simulink model "pd_controller_j2n6s300"  (R2022a)
settings: Solver=ode4  StartTime=0.0  StopTime=0.2  FixedStep=0.01  RelTol=1e-3  EnableMultiTasking=on
undefined symbols (not defined in the file or in its folder): equation_of_motion
libraries: simulink x6
settings Model: Creator=user  LastModifiedBy=47116
settings SolverCC: AlgebraicLoopSolver=TrustRegion
settings DataIOCC: LimitDataPoints=on  SaveFormat=Array
settings OptimizationCC: LifeSpan=inf
settings DebuggingCC: UnconnectedInputMsg=warning  UnconnectedOutputMsg=warning  UnconnectedLineMsg=warning  SFUnexpectedBacktrackingDiag=warning  SFNoUnconditionalDefaultTransitionDiag=warning  SFExecutionAtInitializationDiag=none  SFMachineParentedDataDiag=warning  ArithmeticOperatorsInVariantConditions=warning
settings HardwareCC: ProdBitPerPointer=32  ProdBitPerSizeT=32  ProdBitPerPtrDiffT=32  ProdLargestAtomicFloat=None  ProdIntDivRoundTo=Undefined  ProdEndianess=Unspecified  ProdWordSize=32  ProdHWDeviceType=32-bit Generic
settings ModelReferenceCC: PropagateSignalLabelsOutOfModel=off
settings SFSimCC: SimUseLocalCustomCode=off  CustomCodeUndefinedFunction=UseInterfaceOnly
settings RTWCC: RTWUseLocalCustomCode=off
settings CodeAppCC: StateflowObjectComments=on
settings GRTTargetCC: TargetLangStandard=C89/C90 (ANSI)
settings ConfigComp: CovMetricSettings=dw  CovSaveCumulativeToWorkspaceVar=on  CovSaveSingleToWorkspaceVar=on  CovExternalEMLEnable=off

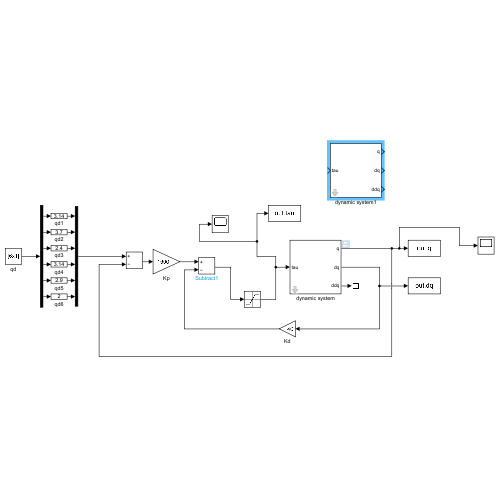
[thumbnail: Simulink's stored preview of the top-level diagram]
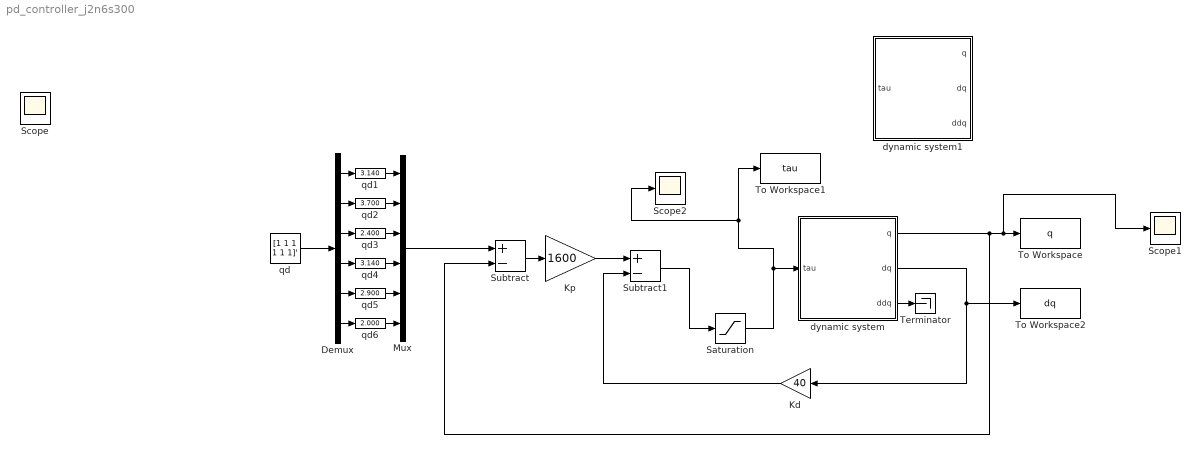
== system pd_controller_j2n6s300 ==
  Demux : Demux  Outputs=6
  Kd : Gain  Gain=40
  Kp : Gain  Gain=1600
  Mux : Mux  Inputs=6
  Saturation : Saturate  UpperLimit=100  LowerLimit=-100
  Scope1 : Scope
  Scope2 : Scope
  Subtract : Sum  Inputs=+-
  Subtract1 : Sum  Inputs=+-
  Terminator : Terminator
  To Workspace : ToWorkspace  VariableName=q  SaveFormat=Timeseries  SampleTime=-1
  To Workspace1 : ToWorkspace  VariableName=tau  SaveFormat=Timeseries  SampleTime=-1
      settings: MaxDataPoints=400
  To Workspace2 : ToWorkspace  VariableName=dq  SaveFormat=Timeseries  SampleTime=-1
  dynamic system : Subsystem  mask{Ts=0.1, phi0=[2.49071610188726;2.06148547305845;-0.729392911612911;-1.96814782905798;1.68425746045805;2.88487012497966], dphi0=[-1.49033763827038;0.446295633676531;7.95542451064005;7.61599085722684;-3.13583558981294;-7.4907928671994]}
      mask prompts: Ts "Sample time"; phi0 "Initial joint positions"; dphi0 "Initial joint velocities"
  dynamic system1 : Subsystem  mask{Ts=0.1, phi0=[2.49071610188726;2.06148547305845;-0.729392911612911;-1.96814782905798;1.68425746045805;2.88487012497966], dphi0=[-1.49033763827038;0.446295633676531;7.95542451064005;7.61599085722684;-3.13583558981294;-7.4907928671994]}
      mask prompts: Ts "Sample time"; phi0 "Initial joint positions"; dphi0 "Initial joint velocities"
  qd : Constant  Value=[1 1 1 1 1 1]'
  qd1 : simulink/Math Operations/Slider Gain  gain=3.140  low=-2  high=3.14
  qd2 : simulink/Math Operations/Slider Gain  gain=3.700  low=-2  high=3.7
  qd3 : simulink/Math Operations/Slider Gain  gain=2.400  low=-2  high=2.4
  qd4 : simulink/Math Operations/Slider Gain  gain=3.140  low=-2  high=3.14
  qd5 : simulink/Math Operations/Slider Gain  gain=2.900  low=-2  high=2.9
  qd6 : simulink/Math Operations/Slider Gain  gain=2.000  low=-3.14  high=2
  Scope : Scope
  wires:
  dynamic system/1(q) -> Subtract/2, Scope1/1, To Workspace/1
  dynamic system/3(ddq) -> Terminator/1
  Demux/2 -> qd2/1
  Demux/4 -> qd4/1
  Demux/6 -> qd6/1
  qd6/1 -> Mux/6
  qd5/1 -> Mux/5
  qd4/1 -> Mux/4
  qd3/1 -> Mux/3
  qd2/1 -> Mux/2
  qd1/1 -> Mux/1
  qd/1 -> Demux/1
  Mux/1 -> Subtract/1
  Demux/3 -> qd3/1
  Demux/5 -> qd5/1
  Subtract1/1 -> Saturation/1
  Demux/1 -> qd1/1
  dynamic system/2(dq) -> To Workspace2/1, Kd/1
  Kp/1 -> Subtract1/1
  Subtract/1 -> Kp/1
  Kd/1 -> Subtract1/2
  Saturation/1 -> Scope2/1, To Workspace1/1, dynamic system/1(tau)

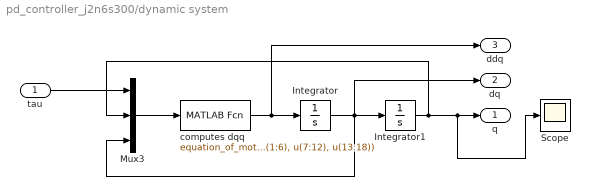
== system pd_controller_j2n6s300/dynamic system ==
  tau : Inport
  Integrator : Integrator  InitialCondition=dphi0
  Integrator1 : Integrator  InitialCondition=phi0
  Mux3 : Mux  Inputs=3
  Scope : Scope
  computes dqq : MATLABFcn  MATLABFcn=equation_of_motion(u(1:6), u(7:12), u(13:18))  OutputDimensions=[6,1]  Output1D=off
  q : Outport
  dq : Outport  Port=2
  ddq : Outport  Port=3
  wires:
  Integrator/1 -> Mux3/3, dq/1, Integrator1/1
  tau/1 -> Mux3/1
  Integrator1/1 -> Mux3/2, Scope/1, q/1
  Mux3/1 -> computes dqq/1
  computes dqq/1 -> ddq/1, Integrator/1

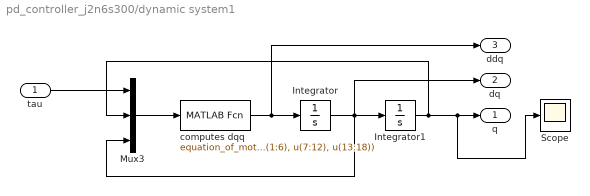
== system pd_controller_j2n6s300/dynamic system1 ==
  tau : Inport
  Integrator : Integrator  InitialCondition=dphi0
  Integrator1 : Integrator  InitialCondition=phi0
  Mux3 : Mux  Inputs=3
  Scope : Scope
  computes dqq : MATLABFcn  MATLABFcn=equation_of_motion(u(1:6), u(7:12), u(13:18))  OutputDimensions=[6,1]  Output1D=off
  q : Outport
  dq : Outport  Port=2
  ddq : Outport  Port=3
  wires:
  Integrator/1 -> Mux3/3, dq/1, Integrator1/1
  tau/1 -> Mux3/1
  Integrator1/1 -> Mux3/2, Scope/1, q/1
  Mux3/1 -> computes dqq/1
  computes dqq/1 -> ddq/1, Integrator/1
